simulink model "model_ciagly"  (R2019b)
settings: Solver=FixedStepAuto  StartTime=0.0  StopTime=20.0  FixedStep=0.01  RelTol=1e-3
settings Model: Creator=szymo  LastModifiedBy=szymo

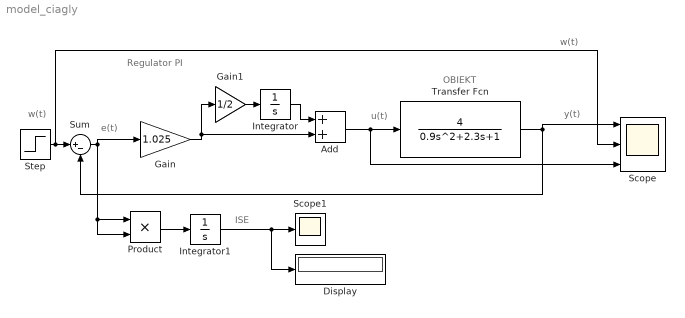
== system model_ciagly ==
  note: w(t)
  note: y(t)
  note: OBIEKT
  note: u(t)
  note: ISE
  note: Regulator PI
  note: e(t)
  note: w(t)
  Add : Sum
  Display : Display
  Gain : Gain  Gain=1.025
  Gain1 : Gain  Gain=1/2
  Integrator : Integrator
  Integrator1 : Integrator
  Product : Product
  Scope : Scope  NumInputPorts=3
  Scope1 : Scope
  Step : Step  Time=0  SampleTime=0
  Sum : Sum  Inputs=|+-
  Transfer Fcn : TransferFcn  Numerator=[4]  Denominator=[0.9 2.3 1]
  wires:
  Step/1 -> Scope/2, Sum/1
  Sum/1 -> Product/2, Product/1, Gain/1
  Gain/1 -> Gain1/1, Add/2
  Gain1/1 -> Integrator/1
  Integrator/1 -> Add/1
  Add/1 -> Scope/3, Transfer Fcn/1
  Transfer Fcn/1 -> Sum/2, Scope/1
  Product/1 -> Integrator1/1
  Integrator1/1 -> Display/1, Scope1/1
